simulink model "Alg_2_112625_Lemon"  (R2025a)
settings: Solver=VariableStepAuto  StartTime=0.0  StopTime=10.0  RelTol=1e-3
libraries: simulink x12, hdlsllib x11, visionhdlio x1
settings Model: Creator=ECE  LastModifiedBy=ECE

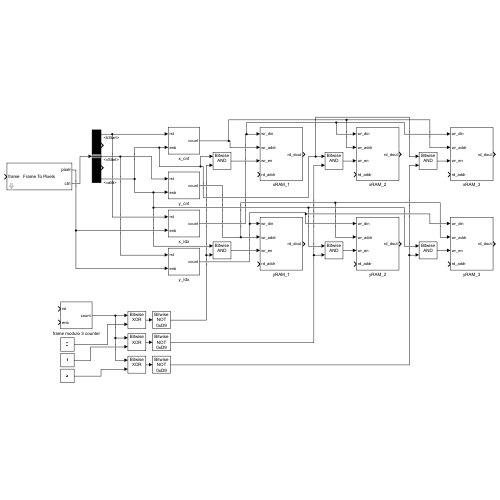
[thumbnail: Simulink's stored preview of the top-level diagram]
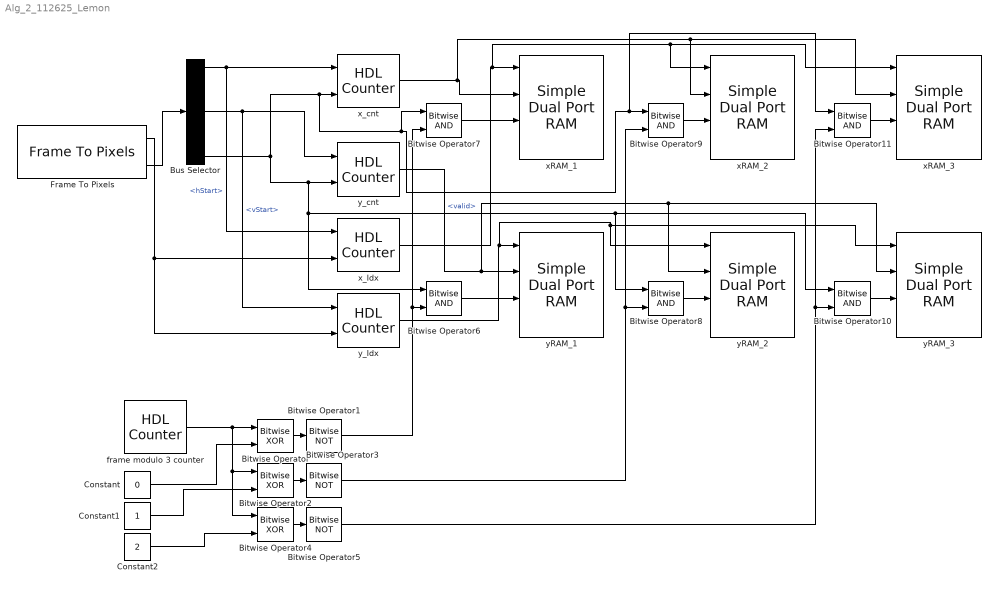
== system Alg_2_112625_Lemon ==
  Bitwise Operator : simulink/Logic and Bit Operations/Bitwise Operator  logicop=XOR  UseBitMask=off  NumInputPorts=2  BitMask=bin2dec('11011001')  BitMaskRealWorld=Stored Integer
      settings: LibrarySourceBlock=|
      | hdlsllib/Logic and Bit
      | Operations/Bitwise
      | Operator
  Bitwise Operator1 : simulink/Logic and Bit Operations/Bitwise Operator  logicop=NOT  UseBitMask=on  BitMask=bin2dec('11011001')  BitMaskRealWorld=Stored Integer
      settings: LibrarySourceBlock=|
      | hdlsllib/Logic and Bit
      | Operations/Bitwise
      | Operator
  Bitwise Operator{6..11} (6 alike) : simulink/Logic and Bit Operations/Bitwise Operator  logicop=AND  UseBitMask=off  NumInputPorts=2  BitMask=bin2dec('11011001')  BitMaskRealWorld=Stored Integer
      settings: LibrarySourceBlock=|
      | hdlsllib/Logic and Bit
      | Operations/Bitwise
      | Operator
  Bitwise Operator2 : simulink/Logic and Bit Operations/Bitwise Operator  logicop=XOR  UseBitMask=off  NumInputPorts=2  BitMask=bin2dec('11011001')  BitMaskRealWorld=Stored Integer
      settings: LibrarySourceBlock=|
      | hdlsllib/Logic and Bit
      | Operations/Bitwise
      | Operator
  Bitwise Operator3 : simulink/Logic and Bit Operations/Bitwise Operator  logicop=NOT  UseBitMask=on  BitMask=bin2dec('11011001')  BitMaskRealWorld=Stored Integer
      settings: LibrarySourceBlock=|
      | hdlsllib/Logic and Bit
      | Operations/Bitwise
      | Operator
  Bitwise Operator4 : simulink/Logic and Bit Operations/Bitwise Operator  logicop=XOR  UseBitMask=off  NumInputPorts=2  BitMask=bin2dec('11011001')  BitMaskRealWorld=Stored Integer
      settings: LibrarySourceBlock=|
      | hdlsllib/Logic and Bit
      | Operations/Bitwise
      | Operator
  Bitwise Operator5 : simulink/Logic and Bit Operations/Bitwise Operator  logicop=NOT  UseBitMask=on  BitMask=bin2dec('11011001')  BitMaskRealWorld=Stored Integer
      settings: LibrarySourceBlock=|
      | hdlsllib/Logic and Bit
      | Operations/Bitwise
      | Operator
  Bus Selector : BusSelector  OutputSignals=hStart,hEnd,vStart,vEnd,valid
  Constant : Constant  Value=0
  Constant1 : Constant
  Constant2 : Constant  Value=2
  Frame To Pixels : visionhdlio/Frame To Pixels  NumComponents=1  NumPixels=1  VideoFormat=1080p  ActivePixelsPerLine=1920  ActiveVideoLines=1080  TotalPixelsPerLine=2200  TotalVideoLines=1125  StartingActiveLine=42  FrontPorch=88  SampleTime=0  VideoFormatCache=1080p  ActivePixelsPerLineCache=32  ActiveVideoLinesCache=18  TotalPixelsPerLineCache=42  TotalVideoLinesCache=28  StartingActiveLineCache=6  FrontPorchCache=5
  frame modulo 3 counter : hdlsllib/Sources/HDL Counter  CountType=Count limited  CountInit=0  CountStep=1  CountMax=2  CountFromType=Initial value  CountFrom=0  CountResetPort=on  CountLoadPort=off  CountEnbPort=on  CountDirPort=off  CountHitOutputPort=off  CountDataType=Unsigned  CountWordLen=8  CountFracLen=0  CountSampTime=1
  xRAM_1 : hdlsllib/HDL RAMs/Simple Dual Port RAM  ram_size=8
  xRAM_2 : hdlsllib/HDL RAMs/Simple Dual Port RAM  ram_size=8
  xRAM_3 : hdlsllib/HDL RAMs/Simple Dual Port RAM  ram_size=8
  x_Idx : hdlsllib/Sources/HDL Counter  CountType=Count limited  CountInit=0  CountStep=1  CountMax=1919  CountFromType=Initial value  CountFrom=0  CountResetPort=on  CountLoadPort=off  CountEnbPort=on  CountDirPort=off  CountHitOutputPort=off  CountDataType=Unsigned  CountWordLen=16  CountFracLen=0  CountSampTime=1
  x_cnt : hdlsllib/Sources/HDL Counter  CountType=Count limited  CountInit=0  CountStep=1  CountMax=1919  CountFromType=Initial value  CountFrom=0  CountResetPort=on  CountLoadPort=off  CountEnbPort=on  CountDirPort=off  CountHitOutputPort=off  CountDataType=Unsigned  CountWordLen=16  CountFracLen=0  CountSampTime=1
  yRAM_1 : hdlsllib/HDL RAMs/Simple Dual Port RAM  ram_size=8
  yRAM_2 : hdlsllib/HDL RAMs/Simple Dual Port RAM  ram_size=8
  yRAM_3 : hdlsllib/HDL RAMs/Simple Dual Port RAM  ram_size=8
  y_Idx : hdlsllib/Sources/HDL Counter  CountType=Count limited  CountInit=0  CountStep=1  CountMax=1079  CountFromType=Initial value  CountFrom=0  CountResetPort=on  CountLoadPort=off  CountEnbPort=on  CountDirPort=off  CountHitOutputPort=off  CountDataType=Unsigned  CountWordLen=16  CountFracLen=0  CountSampTime=1
  y_cnt : hdlsllib/Sources/HDL Counter  CountType=Count limited  CountInit=0  CountStep=1  CountMax=1079  CountFromType=Initial value  CountFrom=0  CountResetPort=on  CountLoadPort=off  CountEnbPort=on  CountDirPort=off  CountHitOutputPort=off  CountDataType=Unsigned  CountWordLen=16  CountFracLen=0  CountSampTime=1
  wires:
  Frame To Pixels/2 -> Bus Selector/1
  Bus Selector/5 -> Bitwise Operator10/1, Bitwise Operator8/1, Bitwise Operator6/1, y_cnt/2, Bitwise Operator11/1, Bitwise Operator9/1, Bitwise Operator7/1, x_cnt/2  "<valid>"
  Bus Selector/1 -> x_Idx/1, x_cnt/1  "<hStart>"
  Bus Selector/3 -> y_Idx/1, y_cnt/1  "<vStart>"
  x_cnt/1 -> xRAM_3/2, xRAM_2/2, xRAM_1/2
  Frame To Pixels/1 -> y_Idx/2, x_Idx/2
  x_Idx/1 -> xRAM_3/1, xRAM_2/1, xRAM_1/1
  y_cnt/1 -> yRAM_3/2, yRAM_2/2, yRAM_1/2
  y_Idx/1 -> yRAM_3/1, yRAM_2/1, yRAM_1/1
  Bitwise Operator/1 -> Bitwise Operator1/1
  frame modulo 3 counter/1 -> Bitwise Operator4/1, Bitwise Operator2/1, Bitwise Operator/1
  Bitwise Operator2/1 -> Bitwise Operator3/1
  Bitwise Operator4/1 -> Bitwise Operator5/1
  Constant/1 -> Bitwise Operator/2
  Constant1/1 -> Bitwise Operator2/2
  Constant2/1 -> Bitwise Operator4/2
  Bitwise Operator1/1 -> Bitwise Operator7/2, Bitwise Operator6/2
  Bitwise Operator6/1 -> yRAM_1/3
  Bitwise Operator7/1 -> xRAM_1/3
  Bitwise Operator8/1 -> yRAM_2/3
  Bitwise Operator9/1 -> xRAM_2/3
  Bitwise Operator3/1 -> Bitwise Operator8/2, Bitwise Operator9/2
  Bitwise Operator11/1 -> xRAM_3/3
  Bitwise Operator10/1 -> yRAM_3/3
  Bitwise Operator5/1 -> Bitwise Operator10/2, Bitwise Operator11/2
